simulink model "THE_3DOF_VESSEL"  (R2022a)
settings: Solver=VariableStepAuto  StartTime=0.0  StopTime=500.0  RelTol=1e-3
libraries: mssSimulink x1
settings Model: Creator=quanv  LastModifiedBy=quanv

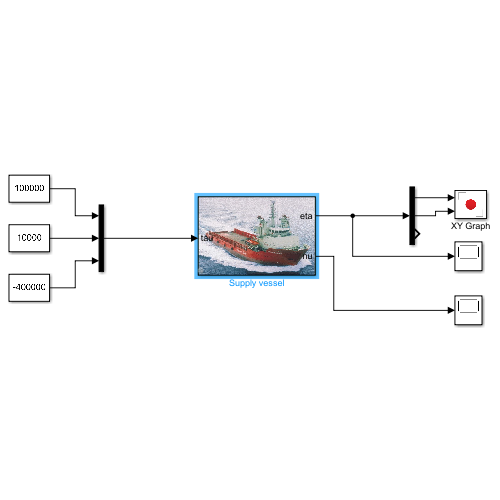
[thumbnail: Simulink's stored preview of the top-level diagram]
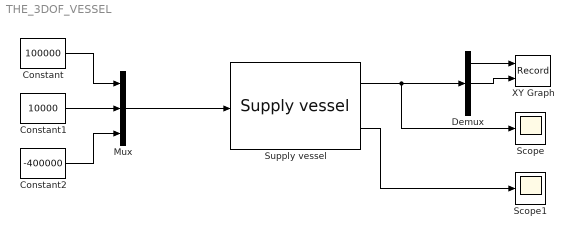
== system THE_3DOF_VESSEL ==
  Constant : Constant  Value=100000
  Constant1 : Constant  Value=10000
  Constant2 : Constant  Value=-400000
  Demux : Demux  Outputs=3
  Mux : Mux  Inputs=3
  Scope : Scope
  Scope1 : Scope
  Supply vessel : mssSimulink/Marine craft models/Supply vessel  D=[5.0242e4 0 0; 0 2.7229e5 -4.3933e6; 0 -4.3933e6 4.1894e8]  Minv=inv( [5.3122e6 0 0; 0 8.2831e6 0; 0 0 3.7454e9] )
  XY Graph : Record  FileSettingsInternal="{\"entries\":[{\"content\":{\"excelSettings\":{\"content\":{},\"type\":\"Streamout.ExcelSettings\"}},\"type\":\"Streamout.FileSettingStorage\",\"uuid\":\"a7829d60-ee65-4f67-ae49-ce969c2049cb\"}],\"packageUris\":[\"http://schema.mathworks.com/mf0/streamout_blocks/R2020a\"],\"version\":\"1.0\"}"  Layout=[1 1]  SignalsInternal="{\"entries\":[{\"content\":{\"signals\":[{\"content\":{\"blockPath\":[\"untitled/XY Graph\"],\"channel\":[],\"dimensions\":[1],\"domain\":\"untitled/XY Graph\",\"lineColor\":\"#a2142f\",\"plots\":[1],\"port\":1,\"sid\":[\"\"],\"signalID\":145,\"signalName\":\"Demux:1\"},\"type\":\"RecordBlkView.Signal\",\"uuid\":\"b2e9851a-9afe-4760-86d7-6d50d73f74c5\"},{\"content\":{\"blockPath\":[\"untitled/XY Graph\"],\"channel\":[],\"dimensions\":[1],\"domain\":\"untitled/XY Graph\",\"lineColor\":\"#139fff\",\"plots\":[1],\"port\":2,\"sid\":[\"\"],\"signalID\":149,\"signalName\":\"Demux:2\"},\"type\":\"RecordBlkView.Signal\",\"uuid\":\"f17f4181-4013-4bd5-9d38-656253a31618\"}]},\"type\":\"RecordBlkView.InputSignals\",\"uuid\":\"5f4f60c1-2b72-432c-9f44-d82ca6c80178\"}],\"packageUris\":[\"http://schema.mathworks.com/mf0/streamout_blocks/R2020a\"],\"version\":\"1.0\"}"  VisualizationBindings="{\"xyplotplugin\":{\"info\":[{\"series\":[{\"bindingParametersList\":[{\"parameter\":\"X-Axis\",\"signalID\":145,\"signalName\":\"Demux:1\"},{\"parameter\":\"Y-Axis\",\"signalID\":149,\"signalName\":\"Demux:2\"}],\"seriesID\":9451}],\"subplotID\":1}]}}"  CompatibilityTag=XY
  wires:
  Mux/1 -> Supply vessel/1
  Constant/1 -> Mux/1
  Constant1/1 -> Mux/2
  Constant2/1 -> Mux/3
  Supply vessel/1 -> Scope/1, Demux/1
  Demux/1 -> XY Graph/1
  Demux/2 -> XY Graph/2
  Supply vessel/2 -> Scope1/1
